simulink model "Test_Harness_v2_3"  (R2023b)
settings: Solver=FixedStepAuto  StartTime=0.0  StopTime=40  RelTol=1e-3  EnableMultiTasking=on
libraries: simulink x2, legoev3lib x2, SignalEditorBlockLib x1
settings Model: ExtModeBatchMode=on  ExtModeTrigDuration=2  Creator=Krish  LastModifiedBy=Krish
settings SolverCC: PositivePriorityOrder=on  AutoInsertRateTranBlk=on
settings OptimizationCC: EnhancedBackFolding=on  PassReuseOutputArgsAs=Individual arguments  ZeroExternalMemoryAtStartup=off  ZeroInternalMemoryAtStartup=off  MaxStackSize=64  OptimizeBlockOrder=speed  DifferentSizesBufferReuse=on  OptimizationCustomize=off  EfficientTunableParamExpr=on
settings DebuggingCC: ParameterTunabilityLossMsg=error
settings HardwareCC: ProdBitPerPointer=32  ProdBitPerSizeT=32  ProdBitPerPtrDiffT=32  ProdLargestAtomicInteger=Long  ProdWordSize=32  ProdHWDeviceType=ARM Compatible->ARM 9
settings SFSimCC: MATLABDynamicMemAlloc=off
settings RTWCC: Description=Embedded Coder  SystemTargetFile=ert.tlc  HardwareBoard=LEGO MINDSTORMS EV3  TLCOptions="-aInlineSetEventsForThisBaseRateFcn=TLC_FALSE -aSuppressMultiTaskScheduler=TLC_FALSE  -aRateBasedStepFcn=0"  TemplateMakefile=ert_default_tmf  Toolchain=Sourcery G++ Lite v2009q3
settings CodeAppCC: ForceParamTrailComments=on  IgnoreCustomStorageClasses=off  OperatorAnnotations=on  SimulinkDataObjDesc=on  SFDataObjDesc=on  InsertBlockDesc=on
settings ERTTargetCC: SupportContinuousTime=on  SupportVariableSizeSignals=on  ExtModeTransport=2  ExtModeStaticAlloc=on  ExtModeMexFile=ext_xcp  ExtModeIntrfLevel=Level2 - Open

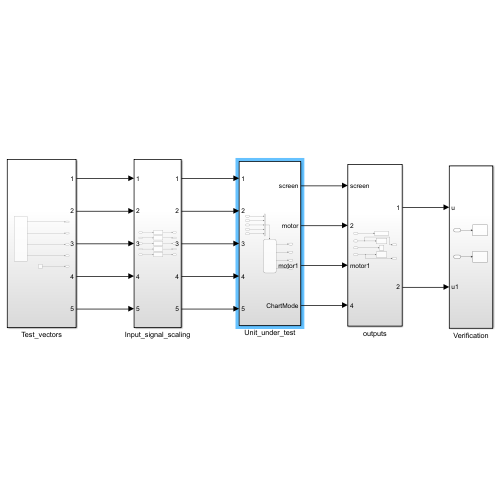
[thumbnail: Simulink's stored preview of the top-level diagram]
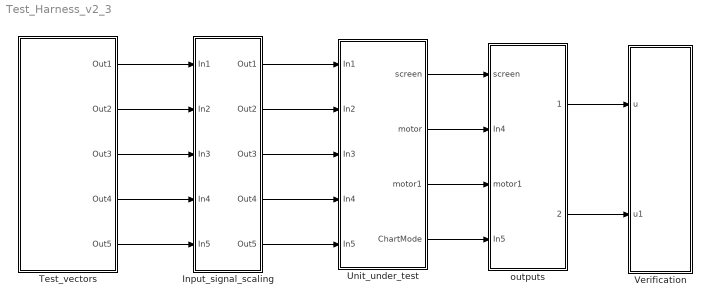
== system Test_Harness_v2_3 ==
  Input_signal_scaling : Subsystem
  Test_vectors : Subsystem
  Unit_under_test : Subsystem
  Verification : Subsystem
  outputs : Subsystem
  wires:
  Unit_under_test/1(screen) -> outputs/1(screen)
  Unit_under_test/2(motor) -> outputs/2(In4)
  Unit_under_test/3(motor1) -> outputs/3(motor1)
  Unit_under_test/4(ChartMode) -> outputs/4(In5)
  Test_vectors/1(Out1) -> Input_signal_scaling/1(In1)
  Test_vectors/2(Out2) -> Input_signal_scaling/2(In2)
  Test_vectors/3(Out3) -> Input_signal_scaling/3(In3)
  Test_vectors/4(Out4) -> Input_signal_scaling/4(In4)
  Test_vectors/5(Out5) -> Input_signal_scaling/5(In5)
  Input_signal_scaling/1(Out1) -> Unit_under_test/1(In1)
  Input_signal_scaling/2(Out2) -> Unit_under_test/2(In2)
  Input_signal_scaling/3(Out3) -> Unit_under_test/3(In3)
  Input_signal_scaling/4(Out4) -> Unit_under_test/4(In4)
  Input_signal_scaling/5(Out5) -> Unit_under_test/5(In5)
  outputs/1(Outport) -> Verification/1(u)
  outputs/2(Outport1) -> Verification/2(u1)

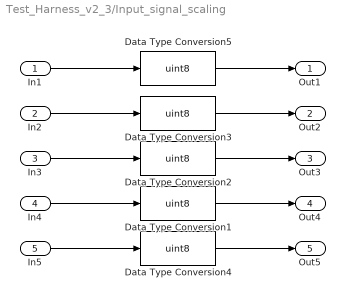
== system Test_Harness_v2_3/Input_signal_scaling ==
  In1 : Inport
  In2 : Inport  Port=2
  In3 : Inport  Port=3
  In4 : Inport  Port=4
  In5 : Inport  Port=5
  Data Type Conversion{1..5} (5 alike) : DataTypeConversion  OutDataTypeStr=uint8  SaturateOnIntegerOverflow=off  RndMeth=Floor
  Out1 : Outport
  Out2 : Outport  Port=2
  Out3 : Outport  Port=3
  Out4 : Outport  Port=4
  Out5 : Outport  Port=5
  wires:
  Data Type Conversion2/1 -> Out3/1
  In5/1 -> Data Type Conversion4/1
  Data Type Conversion3/1 -> Out2/1
  In1/1 -> Data Type Conversion5/1
  Data Type Conversion5/1 -> Out1/1
  Data Type Conversion4/1 -> Out5/1
  In2/1 -> Data Type Conversion3/1
  In3/1 -> Data Type Conversion2/1
  In4/1 -> Data Type Conversion1/1
  Data Type Conversion1/1 -> Out4/1

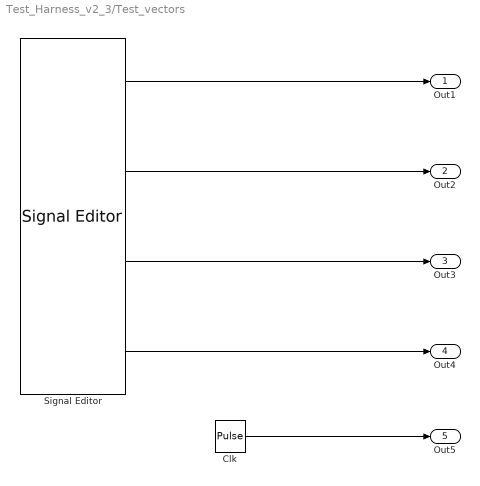
== system Test_Harness_v2_3/Test_vectors ==
  Clk : DiscretePulseGenerator  Period=10  PulseWidth=2
  Signal Editor : SignalEditorBlockLib/Signal Editor  FileName=Signal_source.mat  ActiveScenario=Scenario  ActiveSignal=ExtPushBtn  IsBus=off  OutputBusObjectStr=Bus: BusObject  SampleTime=0  Interpolate=off  ZeroCross=off  OutputAfterFinalValue=Setting to zero  Unit=inherit  PreserveSignalName=on  ApplySigPropsToAllScenarios=on  ApplySigPropsToAllSignals=on
  Out1 : Outport
  Out2 : Outport  Port=2
  Out3 : Outport  Port=3
  Out4 : Outport  Port=4
  Out5 : Outport  Port=5
  wires:
  Signal Editor/1 -> Out1/1
  Signal Editor/2 -> Out2/1
  Signal Editor/3 -> Out3/1
  Signal Editor/4 -> Out4/1
  Clk/1 -> Out5/1

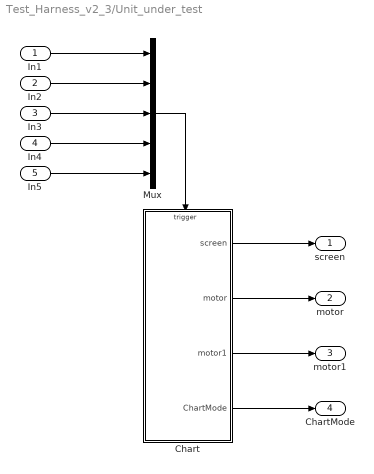
== system Test_Harness_v2_3/Unit_under_test ==
  In1 : Inport
  In2 : Inport  Port=2
  In3 : Inport  Port=3
  In4 : Inport  Port=4
  In5 : Inport  Port=5
  Chart : Stateflow chart  TreatAsAtomicUnit=on
  Mux : Mux  Inputs=5
  screen : Outport
  motor : Outport  Port=2
  motor1 : Outport  Port=3
  ChartMode : Outport  Port=4
  wires:
  Chart/2(motor) -> motor/1
  Mux/1 -> Chart/Trigger
  Chart/4(ChartMode) -> ChartMode/1
  In2/1 -> Mux/2
  In1/1 -> Mux/1
  Chart/1(screen) -> screen/1
  Chart/3(motor1) -> motor1/1
  In4/1 -> Mux/4
  In3/1 -> Mux/3
  In5/1 -> Mux/5

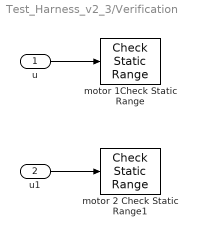
== system Test_Harness_v2_3/Verification ==
  u : Inport
  u1 : Inport  Port=2
  motor 1Check Static Range : simulink/Model Verification/Check  Static Range  Description=0 <= u <= 100  max=100  max_included=on  min=0  min_included=on  enabled=on  callback=Signal_fail  stopWhenAssertionFail=on  export=off  icon=graphic
  motor 2 Check Static Range1 : simulink/Model Verification/Check  Static Range  Description=0 <= u <= 100  max=100  max_included=on  min=0  min_included=on  enabled=on  callback=Signal_fail  stopWhenAssertionFail=on  export=off  icon=graphic
  wires:
  u/1 -> motor 1Check Static Range/1
  u1/1 -> motor 2 Check Static Range1/1

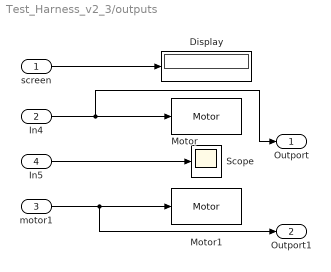
== system Test_Harness_v2_3/outputs ==
  screen : Inport
  In4 : Inport  Port=2
  motor1 : Inport  Port=3
  In5 : Inport  Port=4
  Display : Display
      settings: Format=long_e
  Motor : legoev3lib/Motor  sportNumber=A  sstopAction=Brake
  Motor1 : legoev3lib/Motor  sportNumber=B  sstopAction=Brake
  Scope : Scope
  Outport : Outport
  Outport1 : Outport  Port=2
  wires:
  In4/1 -> Outport/1, Motor/1
  In5/1 -> Scope/1
  screen/1 -> Display/1
  motor1/1 -> Outport1/1, Motor1/1

== stateflow chart Test_Harness_v2_3/Unit_under_test/Chart ==
  settings: executeAtInitialization=1
  state TurnOffConfirm
    entry:
    screen = "confirm";
  state Off
    entry:
    motor=0;
    during:
    screen="Stopped";
  state On1
    entry:
    motor =100;
    motor1=100;
    during:
    screen="Running";
  state TurnOnConfirm
    entry:
    screen = "confirm?";
  state OFF2
    during:
    motor=0;
    motor1=0;
  state EmergencySTOP
    entry:
    motor=0;
    during:
    screen="EmergencySTOP";
  state mid_state
  TurnOffConfirm -> (junction 50) [order 2] : confirm{screen="confrimed"}
  (junction 50) -> Off
  TurnOffConfirm -> On1 [order 1] : deny{screen="denided"}
  On1 -> TurnOffConfirm [order 2] : Center_btn_pressed
  (default) -> Off
  TurnOnConfirm -> Off [order 3] : confirm{screen="confrimed"}
  On1 -> TurnOnConfirm [order 3] : Center_btn_pressed
  TurnOnConfirm -> Off [order 2] : deny{screen="denied"}
  On1 -> OFF2 [order 4] : after(2.1,sec)
  Off -> TurnOnConfirm : Center_btn_pressed
  TurnOnConfirm -> On1 [order 1] : confirm{screen="confrimed"}
  (junction 101) -> On1
  On1 -> (junction 83) [order 1]
  (junction 83) -> EmergencySTOP : e_btnPressed{screen="Emergency Stop"}
  EmergencySTOP -> (junction 90)
  (junction 91) -> EmergencySTOP
  (junction 90) -> mid_state : e_btnPressed
  mid_state -> (junction 101) [order 2] : e_btnPressed
  mid_state -> (junction 91) [order 1] : after(4,sec)
  data: screen output string =0; motor output =0; motor1 output; ChartMode output Enum: ChartModeType
  events: e_btnPressed input RISING_EDGE_EVENT; Center_btn_pressed input RISING_EDGE_EVENT; confirm input RISING_EDGE_EVENT; deny input RISING_EDGE_EVENT; clock input RISING_EDGE_EVENT
